simulink model "bangbang"  (R2020b)
settings: Solver=VariableStepAuto  StartTime=0.0  StopTime=1000  RelTol=1e-3
settings Model: Creator=Javad  LastModifiedBy=Javad

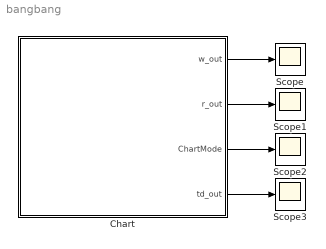
== system bangbang ==
  Chart : Stateflow chart  TreatAsAtomicUnit=on
  Scope{,1..3} (4 alike) : Scope
  wires:
  Chart/1(w_out) -> Scope/1
  Chart/2(r_out) -> Scope1/1
  Chart/3(ChartMode) -> Scope2/1
  Chart/4(td_out) -> Scope3/1

== stateflow chart bangbang/Chart ==
  settings: updateMethod=CONTINUOUS
  state Q1
    du:
    w_dot=-r/10;
    r_dot=0.5*rand(1);
    w_out=w;
    r_out=r;
    td_out=td;
  state Q2
    du:
    w_dot=5/10*(1/2+0.5*sign(t-td-T))-r/10;
    r_dot=0.5*rand(1);
    w_out=w;
    r_out=r;
    td_out=td;
  state Q3
    du:
    w_dot=-r/10;
    r_dot=0;
    w_out=w;
    r_out=r;
    td_out=td;
  state Q4
    du:
    w_dot=5/10*(1/2+0.5*sign(t-td-T))-r/10;
    r_dot=0;
    w_out=w;
    r_out=r;
    td_out=td;
  (default) -> Q1 : {w=10
      | r=0
      | td=0;
      | T=5;}
  Q1 -> Q2 [order 2] : [w<=3.0]
  Q2 -> Q1 [order 2] : [w>=20]
  Q1 -> Q3 [order 1] : [r>=4]{r=4;}
  Q2 -> Q4 [order 1] : [r>=4]{r=4;td=t+T-0.01}
  Q3 -> Q4 : [w<=3.0]{td=t}
  Q4 -> Q3 : [w>=20]
  data: w_out output; r_out output; td local; T local; r local; w local; ChartMode output Enum: ChartModeType; td_out output
  data r settings: updateMethod=SF_CONTINUOUS_TIME_DATA
  data w settings: updateMethod=SF_CONTINUOUS_TIME_DATA
